simulink model "RefGen"  (Simulink 9.3)
settings: Solver=ode4  StartTime=0.0  StopTime=200  FixedStep=1  MaxStep=1  EnableMultiTasking=on
values from neighbouring files (symbols this model uses):
  car = vehicleData    [RunEngine.m]
settings Model: Creator=nkymark  LastModifiedBy=markng
settings SolverCC: MaxConsecutiveMinStep=100  ZeroCrossControl=DisableAll  SolverResetMethod=Robust
settings DataIOCC: ExternalInput=[t,u]  SaveOutput=off  SaveTime=off
settings DebuggingCC: AllowSymbolicDim=off  PregeneratedLibrarySubsystemCodeDiagnostic=none
settings SFSimCC: SimParseCustomCode=off
settings GRTTargetCC: GeneratePreprocessorConditionals=Disable all

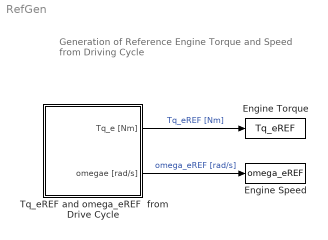
== system RefGen ==
  note: Generation of Reference
      | Engine Torque and Speed from
      | Driving Cycle
  Engine Speed : ToWorkspace  VariableName=omega_eREF  SaveFormat=Timeseries  SampleTime=-1
  Engine Torque : ToWorkspace  VariableName=Tq_eREF  SaveFormat=Timeseries  SampleTime=-1
  Tq_eREF and omega_eREF  from Drive Cycle : Subsystem
  wires:
  Tq_eREF and omega_eREF  from Drive Cycle/1(Tq_e [Nm]) -> Engine Torque/1  "Tq_eREF [Nm]"
  Tq_eREF and omega_eREF  from Drive Cycle/2(omegae [rad/s]) -> Engine Speed/1  "omega_eREF [rad/s]"

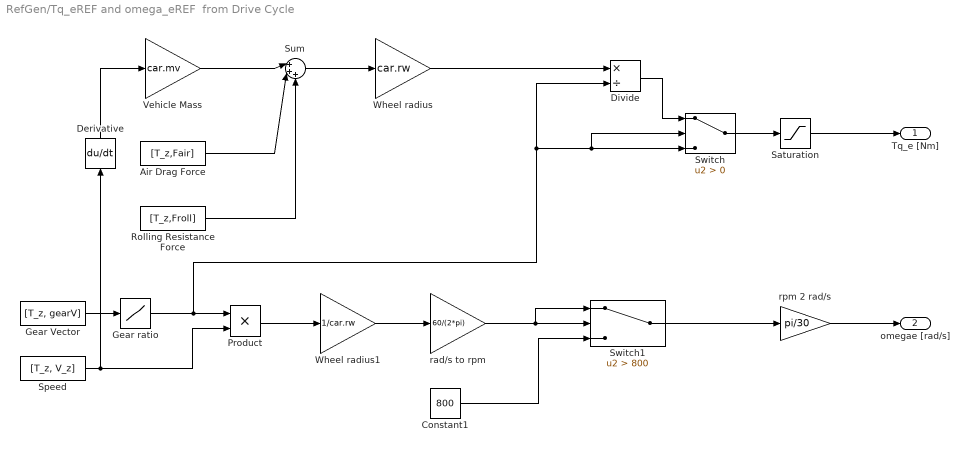
== system RefGen/Tq_eREF and omega_eREF  from Drive Cycle ==
  Air Drag Force : FromWorkspace  VariableName=[T_z,Fair]  SampleTime=0
  Constant1 : Constant  Value=800
  Derivative : Derivative
  Divide : Product  Inputs=*/
  Gear Vector : FromWorkspace  VariableName=[T_z, gearV]  SampleTime=0
  Gear ratio : Lookup  InputValues=[0:8]  Table=[0 14.5635 8.4024 5.4093 4.0417 3.3871 2.7740 2.2442 1.8669]  SaturateOnIntegerOverflow=on
  Product : Product
  Rolling Resistance Force : FromWorkspace  VariableName=[T_z,Froll]  SampleTime=0
  Saturation : Saturate  UpperLimit=car.T_e_max  LowerLimit=1
  "Speed " : FromWorkspace  VariableName=[T_z, V_z]  SampleTime=0
  Sum : Sum  Inputs=|+++
  Switch : Switch  Criteria=u2 > Threshold
  Switch1 : Switch  Criteria=u2 > Threshold  Threshold=800
  Vehicle Mass : Gain  Gain=car.mv
  Wheel radius : Gain  Gain=car.rw
  Wheel radius1 : Gain  Gain=1/car.rw
  rad/s to rpm : Gain  Gain=60/(2*pi)
  rpm 2 rad/s : Gain  Gain=pi/30  SaturateOnIntegerOverflow=on  OutDataTypeStr=Inherit: Same as input  ParamDataTypeStr=Inherit: Same as input
  Tq_e [Nm] : Outport
  omegae [rad/s] : Outport  Port=2
  wires:
  Rolling Resistance Force/1 -> Sum/3
  Gear Vector/1 -> Gear ratio/1
  Vehicle Mass/1 -> Sum/1
  Saturation/1 -> Tq_e [Nm]/1
  Switch/1 -> Saturation/1
  rad/s to rpm/1 -> Switch1/1, Switch1/2
  Constant1/1 -> Switch1/3
  Wheel radius1/1 -> rad/s to rpm/1
  Product/1 -> Wheel radius1/1
  Switch1/1 -> rpm 2 rad/s/1
  Gear ratio/1 -> Product/1, Switch/2, Switch/3, Divide/2
  Derivative/1 -> Vehicle Mass/1
  Air Drag Force/1 -> Sum/2
  Divide/1 -> Switch/1
  Sum/1 -> Wheel radius/1
  Wheel radius/1 -> Divide/1
  "Speed "/1 -> Product/2, Derivative/1
  rpm 2 rad/s/1 -> omegae [rad/s]/1
